simulink model "amplifierboard"  (R2020b)
settings: Solver=FixedStepDiscrete  StartTime=0.0  StopTime=2  FixedStep=0.01  RelTol=1e-3
InitFcn:
  | mbd_s32k_consistency_checks(bdroot(gcs));
undefined symbols (not defined in the file): AutoLowerVal, AutoRaiseVal, HoldVal, LED_En, LED_Off, LED_On, Logic_High, Logic_Low, LQFP, ManualLowerVal, ManualRaiseVal, PWRWNDW_CHDLCK, sC_bool_PWMEN, sC_cnt_FWSetting, sC_cnt_Mtr_DrvNo_HB, sC_cnt_PWMHB1to4, sC_cnt_PWMHB5to8, sC_cnt_TargetSlowRange, sC_pct_ManualMax, sC_pct_RampDwn, sC_pct_RampUp, sC_pct_StartPWM, sC_pct_Targetmax, SwitchPackRangeOffset, Threshold_Value, Tolerant_Time
libraries: mbd_s32k1xx_ec_toolbox x205, simulink x59, canmsglib x19, Filter x15, wndwcmd x3
(part 6 of 6)

== stateflow chart amplifierboard/Motor_Control/Motor_Control/Chart ==
  note: SPI Format:
      |
      | SPI Command:
      | Bit
      | B15
      | B14
      | B13
      | B12
      | B11
      | B10
      | B9
      | B8
      | B7
      | B6
      | B5
      | B4
      | B3
      | B2
      | B1
      | B0
      |
      | Data
      | 0
      | R/W
      | A5
      | A4
      | A3
      | A2
      | A1
      | A0
      | D7
      | D6
      | D5
      | D4
      | D3
      | D2
      | D1
      | D0
      |
      | Description
      | Default
      | WRITE =0
      | Register Address
      | Data
      |
      | Bit
      | B15
      | B14
      | B13
      | B12
      | B11
      | B10
      | B9
      | B8
      | B7
      | B6
      | B5
      | B4
      | B3
      | B2
      | B1
      | B0
      |
      | Data
      | 1
      | 1
      | FAULT
      | WARN
      | DS_GS
      | UV
      | OV
      | OT_WD_AGD
      | D7
      | D6
      | D5
      | D4
      | D3
      | D2
      | D1
      | D0
      |
      | Description
      | Default
      | Default
      | Fault
      | indicator
      | Warning
      | Indicator
      | Logic OR
      | of Vds and
      | Vgs fault indicator
      | UnderVoltage
      | indicator
      | OverVoltage
      | indicator
      | Logic OR of OTW,
      | OTSD,WD_FLT,
      | IDIR_WARN,
      | PDCHR_WARN,
      | and STC_WARN
      | indicators
      | Report
      |
      | Important Commands:
      |
      | Command name
      | as per datasheet
      | Command use
      | Address
      | (6 bits)
      | B7
      | B6
      | B5
      | B4
      | B3
      | B2
      | B1
      | B0
      |
      | IC_CTRL1
      | Control register for driver
      | and diagnostic enable, SPI lock and clear fault
      | 0x07
      | EN_DRV
      | 0 = gate drv output disabled
      | 1 = gate drv output enabled
      |
      | EN_OLSC
      | 0 = disable
      | 1 = enable
      | RESERVED
      | (00)
      | LOCK
      | 011 = Unlock all ctrl reg
      | 110 = lock
      | CLR_FLT
      | 0 = Default
      | 1 = clear fault
      |
      | IC_CTRL2
      | Control register for pin mode, charge pump
      | mode, and watchdog
      | 0x08
      | DIS_SSC
      | Spread Spectrum clocking
      | 0 = EN, 1 = ~EN
      |
      | DRVOff_nFLT
      | Sets DRVOff/nFLT
      | multi-fn pin mode
      | 0 = pin as DRVoff
      | 1 = pin as nFLT
      | Charge pump op mode
      | 00 = auto switch bw modes
      | 01 = always doubler
      | 10 = always tripler
      | 11 = Reserved
      | WD_EN
      | 0 = disabled
      | 1 = enabled
      | Watchdog flt mode
      |
      | WatchDog timer
      | 0 = 4 - 40ms
      | 1 = 10- 100ms
      | WatchDog Reset
      | 0 is default.
      | Invert to restart
      | timer
      |
      | VDS_CTRL1
      | Control register to set Vds overcurrent TH on HB 1& 2
      | 0x1F
      | HB-1; Range from 0.06V to 2V (Refer to page 88 on data sheet) (1101 = 1V)
      | HB-2; Range from 0.06V to 2V (Refer to page 88 on data sheet) (1101 = 1V)
      |
      | VDS_CTRL2
      | Control register to set Vds overcurrent TH on HB 3& 4
      | 0x20
      | HB-3; Range from 0.06V to 2V (Refer to page 88 on data sheet) (1101 = 1V)
      | HB-4; Range from 0.06V to 2V (Refer to page 88 on data sheet) (1101 = 1V)
      |
      | VDS_CTRL3
      | Control register to set Vds overcurrent TH on HB 5& 6
      | 0x21
      | HB-5; Range from 0.06V to 2V (Refer to page 88 on data sheet) (1101 = 1V)
      | HB-6; Range from 0.06V to 2V (Refer to page 88 on data sheet) (1101 = 1V)
      |
      | VDS_CTRL4
      | Control register to set Vds overcurrent TH on HB 7& 8
      | 0x22
      | HB-7; Range from 0.06V to 2V (Refer to page 88 on data sheet) (1101 = 1V)
      | HB-8; Range from 0.06V to 2V (Refer to page 88 on data sheet) (1101 = 1V)
      |
      | PWM_CTRL1
      | Control register to map input PWM source for HB 1-4
      | 0x0B
      | HB-1 Setting: 00 = PWM1, 01 = PWM2,
      | 10 = PWM3, 11 = PWM4
      | HB-2 Setting: 00 = PWM1, 01 = PWM2,
      | 10 = PWM3, 11 = PWM4
      | HB-3 Setting: 00 = PWM1, 01 = PWM2,
      | 10 = PWM3, 11 = PWM4
      | HB-4 Setting: 00 = PWM1, 01 = PWM2,
      | 10 = PWM3, 11 = PWM4
      |
      | PWM_CTRL2
      | Control register to map input PWM source for HB 5-8
      | 0x0C
      | HB-5 Setting: 00 = PWM1, 01 = PWM2,
      | 10 = PWM3, 11 = PWM4
      | HB-5 Setting: 00 = PWM1, 01 = PWM2,
      | 10 = PWM3, 11 = PWM4
      | HB-5 Setting: 00 = PWM1, 01 = PWM2,
      | 10 = PWM3, 11 = PWM4
      | HB-5 Setting: 00 = PWM1, 01 = PWM2,
      | 10 = PWM3, 11 = PWM4
      |
      | PWM_CTRL3
      | Control register to select pwm drive mosfet for HB 1-8
      | 0x0D
      | HB-1
      | 0 = High side MOSFET
      | 1 = Low side MOSFET
      | HB-2
      | 0 = High side MOSFET
      | 1 = Low side MOSFET
      | HB-3
      | 0 = High side MOSFET
      | 1 = Low side MOSFET
      | HB-4
      | 0 = High side MOSFET
      | 1 = Low side MOSFET
      | HB-5
      | 0 = High side MOSFET
      | 1 = Low side MOSFET
      | HB-6
      | 0 = High side MOSFET
      | 1 = Low side MOSFET
      | HB-7
      | 0 = High side MOSFET
      | 1 = Low side MOSFET
      | HB-8
      | 0 = High side MOSFET
      | 1 = Low side MOSFET
      |
      | PWM_CTRL4
      | Control register to set HB Freewheeling mode (action taken for back emf when motor stops) - Choose 0 for all
      | (inverted pwm is faster than freewheeling diode)
      | 0x0E
      | HB-1
      | 0 = invert pwm
      | 1 = rely on freewheeling
      | diode
      | HB-2
      | 0 = invert pwm
      | 1 = rely on freewheeling
      | diode
      | HB-3
      | 0 = invert pwm
      | 1 = rely on freewheeling
      | diode
      | HB-4
      | 0 = invert pwm
      | 1 = rely on freewheeling
      | diode
      | HB-5
      | 0 = invert pwm
      | 1 = rely on freewheeling
      | diode
      | HB-6
      | 0 = invert pwm
      | 1 = rely on freewheeling
      | diode
      | HB-7
      | 0 = invert pwm
      | 1 = rely on freewheeling
      | diode
      | HB-8
      | 0 = invert pwm
      | 1 = rely on freewheeling
      | diode
      |
      | BRG_CTRL1
      | Control register to set output state for HB 1-4
      | 0x09
      | HB-1 control:
      | 00 = HI-Z GH1 and GH2 pulldwn
      | 01 = Drive LS. GH1 pullup GH2 pulldown
      | 10 = Drive HS. GH! pulldown GH1 pullup
      | 11 = Input PWM ctrl.
      | HB-2 control:
      | 00 = HI-Z GH1 and GH2 pulldwn
      | 01 = Drive LS. GH1 pullup GH2 pulldown
      | 10 = Drive HS. GH! pulldown GH1 pullup
      | 11 = Input PWM ctrl.
      | HB-3 control:
      | 00 = HI-Z GH1 and GH2 pulldwn
      | 01 = Drive LS. GH1 pullup GH2 pulldown
      | 10 = Drive HS. GH! pulldown GH1 pullup
      | 11 = Input PWM ctrl.
      | HB-4 control:
      | 00 = HI-Z GH1 and GH2 pulldwn
      | 01 = Drive LS. GH1 pullup GH2 pulldown
      | 10 = Drive HS. GH! pulldown GH1 pullup
      | 11 = Input PWM ctrl.
      |
      | BRG_CTRL2
      | Control register to set output state fot HB 5-8
      | 0x0A
      | HB-5 control:
      | 00 = HI-Z GH1 and GH2 pulldwn
      | 01 = Drive LS. GH1 pullup GH2 pulldown
      | 10 = Drive HS. GH! pulldown GH1 pullup
      | 11 = Input PWM ctrl.
      | HB-6 control:
      | 00 = HI-Z GH1 and GH2 pulldwn
      | 01 = Drive LS. GH1 pullup GH2 pulldown
      | 10 = Drive HS. GH! pulldown GH1 pullup
      | 11 = Input PWM ctrl.
      | HB-7 control:
      | 00 = HI-Z GH1 and GH2 pulldwn
      | 01 = Drive LS. GH1 pullup GH2 pulldown
      | 10 = Drive HS. GH! pulldown GH1 pullup
      | 11 = Input PWM ctrl.
      | HB-8 control:
      | 00 = HI-Z GH1 and GH2 pulldwn
      | 01 = Drive LS. GH1 pullup GH2 pulldown
      | 10 = Drive HS. GH! pulldown GH1 pullup
      | 11 = Input PWM ctrl.
      |
      | IC_STAT1
      | Status register for global fault and warning indicators
      | (when sending remember to have read/write bit as 1 aka read) and data field should all be zeros
      | 0x00
      | SPI_OK
      | 0 = multiple SCLK FLT
      | 1 = No SPI fault
      | POR
      | 0 = no Power on reset event
      | 1 = Power on reset detected
      | FAULT
      |
      | WARN
      | DS_GS
      | UV
      | OV
      | OT_WD_AGD
  state HB_PWM_Vds_Settingsen_
    en: Drv_idx = 1;
    MotorDriverState=3;
    state PWM_CTRL4
      %Freewheel setup
      en: SendSPI(Drv_idx,[0b00001110, sC_cnt_FWSetting(Drv_idx)]);
      %0b00000000
    state VDS_CTRL1
      %Set HB 1 & 2 to 1V OC Threshold
      en: SendSPI(Drv_idx,[0b00011111, 0b11011101]);
    state VDS_CTRL2
      %Set HB 3 & 4 to 1V OC Threshold
      en:  SendSPI(Drv_idx,[0b00100000, 0b11011101]);
    state VDS_CTRL3
      %Set HB 5 & 6 to 1V OC Threshold
      en: SendSPI(Drv_idx,[0b00100001, 0b11011101]);
    state VDS_CTRL4
      %Set HB 7 & 8 to 1V OC Threshold
      en: SendSPI(Drv_idx,[0b00100010, 0b11011101]);
    state PWM_CTRL1
      %PWM Mapping for HB 1 to 4.
      %HB 1,2 = PWM1; 3,4 = PWM2;
      en: SendSPI(Drv_idx,[0b00001011, sC_cnt_PWMHB1to4(Drv_idx)]);
    state PWM_CTRL2
      %PWM Mapping for HB 5 to 8.
      %HB 5,6 = PWM3; 7,8 = PWM4;
      en: SendSPI(Drv_idx,[0b00001100, sC_cnt_PWMHB5to8(Drv_idx)]);
    (default) -> PWM_CTRL4
    PWM_CTRL4 -> VDS_CTRL1
    VDS_CTRL1 -> VDS_CTRL2
    VDS_CTRL2 -> VDS_CTRL3
    VDS_CTRL3 -> VDS_CTRL4
    VDS_CTRL4 -> HB_PWM_Vds_Settingsen_.PWM_CTRL1
    HB_PWM_Vds_Settingsen_.PWM_CTRL1 -> HB_PWM_Vds_Settingsen_.PWM_CTRL2
    HB_PWM_Vds_Settingsen_.PWM_CTRL2 -> HB_PWM_Vds_Settingsen_ [order 2] : {Drv_idx = Drv_idx + 1;}
        | %Driver index increment
  state Drivers_ON_Init
    en: DRV1_OFF = false;
    en: DRV2_OFF = false;
    du: int_count = int_count + 1;
    MotorDriverState=1;
    %Enable all drivers
  state Disable_WD_and_Clear_Faults
    en: Drv_idx = 1;
    MotorDriverState=2;
    state IC_CTRL2_WDG
      %WatchDog Disable, Setting WD timer to 100ms
      en: SendSPI(Drv_idx,[0b00001000, 0b00000110]);
    state IC_CTRL1
      %Enable Driver, Clear Faults
      en: SendSPI(Drv_idx,[0b00000111, 0b10000111]);
    (default) -> IC_CTRL2_WDG
    IC_CTRL2_WDG -> Disable_WD_and_Clear_Faults.IC_CTRL1
    Disable_WD_and_Clear_Faults.IC_CTRL1 -> Disable_WD_and_Clear_Faults [order 2] : {Drv_idx = Drv_idx + 1;}
        | %Driver index increment
  state Drivers_OFF [commented out]
    en: DRV1_OFF = true;
    en: DRV2_OFF = true;
    en: DRV3_OFF = true;
    du: int_count = int_count + 1;
    %Disable all drivers
  state StatusOut = SendSPI(DriverNo,SPICommand) [function]
  note: ChipSelect
      | Pin
      | Driver
      |
      | PCS0
      | PTD3
      | DRV1
      |
      | PCS2
      | PTA16
      | DRV2
  state Drivers_ON [commented out]
    en: DRV1_OFF = false;
    en: DRV2_OFF = false;
    en: DRV3_OFF = false;
    du: int_count = int_count + 1;
    %Enable all drivers
  state IC_CTRL2_WatchDog
    %Toggle LSB in second byte for WD Reset
    en: Drv_idx = 1;
    en,du: DriverStatus(Drv_idx,:) = SendSPI(Drv_idx,[0b00001000,Drv_WD_Cmd] );
    en,du: FailSafe(Drv_idx) = bitand(DriverStatus(Drv_idx,1),uint8(0b00111111));
    en,du: Drv_idx = Drv_idx + 1;
    MotorDriverState=  4;
  state FailSafe_Clear_Faults
    en: MotorDriverState=5;
    %Clear faults and reassign PWM
    state IC_CTRL1
      %Enable Driver, Clear Faults
      en: SendSPI(Drv_idx,[0b00000111, 0b10000111]);
    state PWM_CTRL1
      %PWM Mapping for HB 1 to 4.
      %HB 1,2 = PWM1; 3,4 = PWM2;
      en: SendSPI(Drv_idx,[0b00001011, sC_cnt_PWMHB1to4(Drv_idx)]);
    state PWM_CTRL2
      %PWM Mapping for HB 5 to 8.
      %HB 5,6 = PWM3; 7,8 = PWM4;
      en: SendSPI(Drv_idx,[0b00001100, sC_cnt_PWMHB5to8(Drv_idx)]);
    (default) -> FailSafe_Clear_Faults.IC_CTRL1
    FailSafe_Clear_Faults.IC_CTRL1 -> FailSafe_Clear_Faults.PWM_CTRL1
    FailSafe_Clear_Faults.PWM_CTRL1 -> FailSafe_Clear_Faults.PWM_CTRL2
  state Motor_Activate_Deactivate
    en: int_Count1 = 0;
    en: Drv_idx = uint8(bitsra(bitand(sC_cnt_Mtr_DrvNo_HB(for_idx),0xF00),8));
    en: HB_A = uint8(bitsra(bitand(sC_cnt_Mtr_DrvNo_HB(for_idx),0x0F0),4));
    en: HB_B = uint8(bitand(sC_cnt_Mtr_DrvNo_HB(for_idx),0x00F));
    du: int_Count1 = int_Count1+1;
    MotorDriverState = 7;
    Motor_Activate_Deactivate -> (junction 180) [order 1]
    (junction 180) -> (junction 182) [order 1] : [int_Count1 == 1]
        | %first command
    (junction 182) -> (junction 221) [order 1] : [aV_int_MotorDir(for_idx)> 0]
        | {Drv_HB_Msg(Drv_idx) = uint16(bitset(Drv_HB_Msg(Drv_idx),(17-(2*HB_A-1)),1));
        | Drv_HB_Msg(Drv_idx) = uint16(bitset(Drv_HB_Msg(Drv_idx),(17-2*HB_A),(1*sC_bool_PWMEN(for_idx))));
        | Drv_HB_Msg(Drv_idx) = uint16(bitset(Drv_HB_Msg(Drv_idx),(17-(2*HB_B-1)),0));
        | Drv_HB_Msg(Drv_idx) = uint16(bitset(Drv_HB_Msg(Drv_idx),(17-2*HB_B),1));}
        | %if positive direction, set pwm on HB_A
    (junction 180) -> (junction 193) [order 2]
    (junction 182) -> (junction 223) [order 2]
    (junction 221) -> (junction 225)
    (junction 223) -> (junction 225) [order 1] : [aV_int_MotorDir(for_idx)< 0]
        | {Drv_HB_Msg(Drv_idx) = uint16(bitset(Drv_HB_Msg(Drv_idx),(17-(2*HB_A-1)),0));
        | Drv_HB_Msg(Drv_idx) = uint16(bitset(Drv_HB_Msg(Drv_idx),(17-2*HB_A),1));
        | Drv_HB_Msg(Drv_idx) = uint16(bitset(Drv_HB_Msg(Drv_idx),(17-(2*HB_B-1)),1));
        | Drv_HB_Msg(Drv_idx) = uint16(bitset(Drv_HB_Msg(Drv_idx),(17-2*HB_B),(1*sC_bool_PWMEN(for_idx))));}
        | %if negative direction, set pwm on HB_B
    (junction 223) -> (junction 228) [order 2]
    (junction 225) -> (junction 230) : {bool_isMoving(for_idx) = true;}
    (junction 228) -> (junction 230) : {Drv_HB_Msg(Drv_idx) = uint16(bitset(Drv_HB_Msg(Drv_idx),(17-(2*HB_A-1)),0));
        | Drv_HB_Msg(Drv_idx) = uint16(bitset(Drv_HB_Msg(Drv_idx),(17-2*HB_A),0));
        | Drv_HB_Msg(Drv_idx) = uint16(bitset(Drv_HB_Msg(Drv_idx),(17-(2*HB_B-1)),0));
        | Drv_HB_Msg(Drv_idx) = uint16(bitset(Drv_HB_Msg(Drv_idx),(17-2*HB_B),0));;
        | bool_isMoving(for_idx) = false;
        | bool_assigned = true;}
        | %if direction is zero, turn off HB_A and HB_B.
    (junction 230) -> (junction 235) [order 2] : {SendSPI(Drv_idx,[0b00001001,uint8(bitsra(bitand(Drv_HB_Msg(Drv_idx),0xFF00),8))]);}
        | %If HB are less than 4, send this command
    (junction 230) -> (junction 235) [order 1] : [HB_A > 4] %if HB are greater than 4, send this command
        | {SendSPI(Drv_idx,[0b00001010,uint8(bitand(Drv_HB_Msg(Drv_idx),0x00FF))]);}
    (junction 235) -> (junction 208)
    (junction 193) -> (junction 211) [order 1] : [int_Count1 == 2]
        | %second command
    (junction 211) -> (junction 208) [order 1] : [aV_int_MotorDir(for_idx) > 0 && sC_bool_PWMEN(for_idx)]
        | {
        | Drv_PWM_Msg(Drv_idx) = uint8(bitset(Drv_PWM_Msg(Drv_idx),(9-HB_A),0));
        | Drv_PWM_Msg(Drv_idx) = uint8(bitset(Drv_PWM_Msg(Drv_idx),(9-HB_B),1));
        | SendSPI(Drv_idx,[0b00001101,Drv_PWM_Msg(Drv_idx)]);
        | bool_assigned = true;
        | }  %send PWM command for HB_A
    (junction 193) -> (junction 218) [order 2]
    (junction 211) -> (junction 212) [order 2]
    (junction 208) -> (junction 209)
    (junction 212) -> (junction 209) [order 1] : [aV_int_MotorDir(for_idx) < 0  && sC_bool_PWMEN(for_idx)]
        | {
        | Drv_PWM_Msg(Drv_idx)  = uint8(bitset(Drv_PWM_Msg(Drv_idx),(9-HB_A),1));
        | Drv_PWM_Msg(Drv_idx) = uint8(bitset(Drv_PWM_Msg(Drv_idx),(9-HB_B),0));
        | SendSPI(Drv_idx,[0b00001101,Drv_PWM_Msg(Drv_idx)]);
        | bool_assigned = true;
        | } %send PWM command for HB_B
    (junction 212) -> (junction 245) [order 2]
    (junction 209) -> (junction 247)
    (junction 245) -> (junction 247) [order 1] : [~sC_bool_PWMEN(for_idx)]
        | {bool_assigned = true;}
        | %PWM disabled
    (junction 245) -> (junction 247) [order 2]
    (junction 247) -> (junction 217)
    (junction 218) -> (junction 217) : %{bool_assigned = true;}
  (default) -> Drivers_ON_Init
  Drivers_ON_Init -> Disable_WD_and_Clear_Faults : [int_count > 10]
      | {int_count= 0;}
  Drivers_OFF -> Drivers_ON [commented out] : [int_count > 10]
      | {int_count = 0;}
  Disable_WD_and_Clear_Faults.IC_CTRL1 -> HB_PWM_Vds_Settingsen_ [order 1] : [Drv_idx == 2]
  HB_PWM_Vds_Settingsen_.PWM_CTRL2 -> (junction 43) [order 1] : [Drv_idx == 2]
  Drivers_ON -> Disable_WD_and_Clear_Faults [commented out] : [int_count > 10]
      | {int_count = 0;}
  (junction 43) -> IC_CTRL2_WatchDog
  (junction 148) -> (junction 43)
  (junction 84) -> IC_CTRL2_WatchDog
  (junction 147) -> (junction 148) : %FailSafe
      | %Reset complete
  (junction 82) -> (junction 84)
  IC_CTRL2_WatchDog -> (junction 133) : [Drv_idx > 2]
      | {Drv_idx = 1;
      |  Drv_WD_Cmd= uint8(bitset(Drv_WD_Cmd,1,~bitget(Drv_WD_Cmd,1)));}
      | %toggle bit for watchdog
  (junction 155) -> FailSafe_Clear_Faults [order 1] : [FailSafe(1)]
      | {Drv_idx = 1;}
      | %Driver 1 Error detected
  (junction 133) -> (junction 155) [order 1] : [any(FailSafe) &&...
      | all(~bool_isMoving)]
      | %any driver in error and all motors idle
  (junction 155) -> (junction 157) [order 2]
  (junction 133) -> (junction 75) [order 2] : {for_idx = 1;
      | bool_assigned = false;}
      | %for loop init
  (junction 157) -> FailSafe_Clear_Faults : [FailSafe(2)]
      | {Drv_idx = 2;}
      | %Driver 2 Error detected
  (junction 75) -> (junction 82) [order 2]
  (junction 87) -> (junction 75) : {for_idx = for_idx + 1;}
      | %for loop
      | % index increment
  (junction 75) -> (junction 80) [order 1] : [for_idx < 7 &&...
      |  ~bool_assigned]
      | %for loop condition
  FailSafe_Clear_Faults.PWM_CTRL2 -> (junction 147)
  (junction 80) -> (junction 100) [order 2] : %default fault
  (junction 100) -> (junction 128) : {Drv_idx = uint8(bitsra(bitand(sC_cnt_Mtr_DrvNo_HB(for_idx),0xF00),8));}
  (junction 80) -> Motor_Activate_Deactivate [order 1] : [(aV_int_MotorDir(for_idx) ~= 0 && ~bool_isMoving(for_idx)) ||...
      |  (aV_int_MotorDir(for_idx) == 0 && bool_isMoving(for_idx))]
      | %motor is inactive and requested to start or
      | %motor is active and requested to stop
  (junction 128) -> (junction 130) [order 1] : [FailSafe(Drv_idx)]
      | {bool_isMoving(for_idx) = false;}
      | %if Failsafe detected for this motor's driver,
      | %reset flag
  (junction 128) -> (junction 130) [order 2]
  Motor_Activate_Deactivate -> (junction 87) [order 1] : [bool_assigned || int_Count1 > 2]
      | %SPI command complete
  (junction 130) -> (junction 102)
  (junction 102) -> (junction 87)
  data: DriverNo function_input uint8 size=1; SPICommand function_input uint8 size=[1 2]; StatusOut function_output; Drv_idx local uint8 size=1 =uint8(0); int_count local =0; DRV1_OFF output boolean size=1 =false; DRV2_OFF output boolean size=1 =false; FailSafe output uint8 size=2 =uint8(zeros(2,1)); bool_isMoving local boolean size=6 =false(6,1); aV_int_MotorDir input int8 size=6; bool_assigned local boolean size=1 =false; sC_cnt_PWMHB1to4 input uint8 size=3; sC_cnt_PWMHB5to8 input uint8 size=3; for_idx local =0; Drv_WD_Cmd local uint8 size=1 =[0b00000110]; int_Count1 local uint8 size=1 =uint8(0); HB_A local uint8 size=1 =uint8(0); HB_B local uint8 size=1 =uint8(0); Drv_PWM_Msg local uint8 size=3 =zeros(3,1,'uint8'); sC_cnt_Mtr_DrvNo_HB input uint16 size=6; Drv_HB_Msg local uint16 size=3 =zeros(3,1,'uint16'); sC_bool_PWMEN input boolean size=6; sC_cnt_FWSetting input uint8 size=3; DriverStatus local uint8 size=[3 2] =uint8(zeros(3,2)); MotorDriverState output uint8 size=1

== matlab function amplifierboard/CAN_Receive_And_Unpack/Subsystem/Chart/ECU_Reset/MATLAB Function ==
function Reset_MCU
%#codegen

if( coder.target( 'Rtw' ) )
    coder.ceval('S32_SCB->AIRCR = S32_SCB_AIRCR_VECTKEY(0x5FA) | S32_SCB_AIRCR_SYSRESETREQ_MASK; //');
end
end
